simulink model "vehicleModel"  (R2022a)
settings: Solver=VariableStepAuto  StartTime=0  StopTime=20  FixedStep=0.01  RelTol=1e-3
InitFcn:
  | lat_sim_parameters
values from neighbouring files (symbols this model uses):
  A = zeros(6)    [find_path_coeffs.m]    (also in getLateralDynamics.m = [0 1 vx 0)
  B = [0; -b1; 0; -b2]    [getLateralDynamics.m]
  C = [1 0 d 0]    [lat_sim_parameters.m]
  Klat = place(A, B, poles)    [lat_sim_parameters.m]    (also in tuneLateralController.m)
  lr = 1.6    [acc_sim_parameters.m]    (also in lat_sim_parameters.m = 2; tuneLateralController.m = 2)
  m = 1575    [acc_sim_parameters.m]    (also in lat_sim_parameters.m = 2000; tuneLateralController.m = 2000)
undefined symbols (not defined in the file or in its folder): vxBar
libraries: autolibshared x1
settings Model: Creator=Fernando VM  LastModifiedBy=fvall
settings SolverCC: AlgebraicLoopSolver=TrustRegion
settings DataIOCC: ExternalInput=[dt, da, dd]  ReturnWorkspaceOutputs=off
settings DebuggingCC: UnconnectedInputMsg=warning  UnconnectedOutputMsg=warning  UnconnectedLineMsg=warning  SFMachineParentedDataDiag=warning  ArithmeticOperatorsInVariantConditions=warning
settings SFSimCC: CustomCodeUndefinedFunction=UseInterfaceOnly

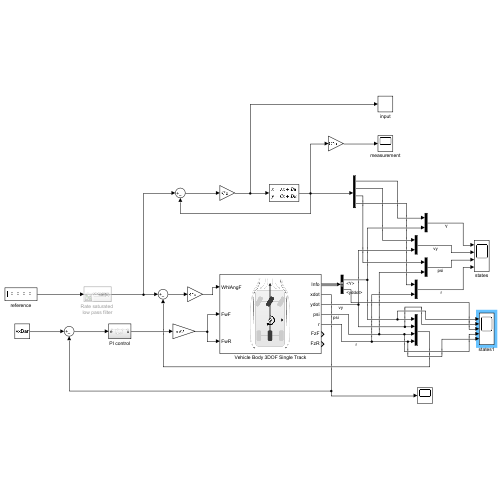
[thumbnail: Simulink's stored preview of the top-level diagram]
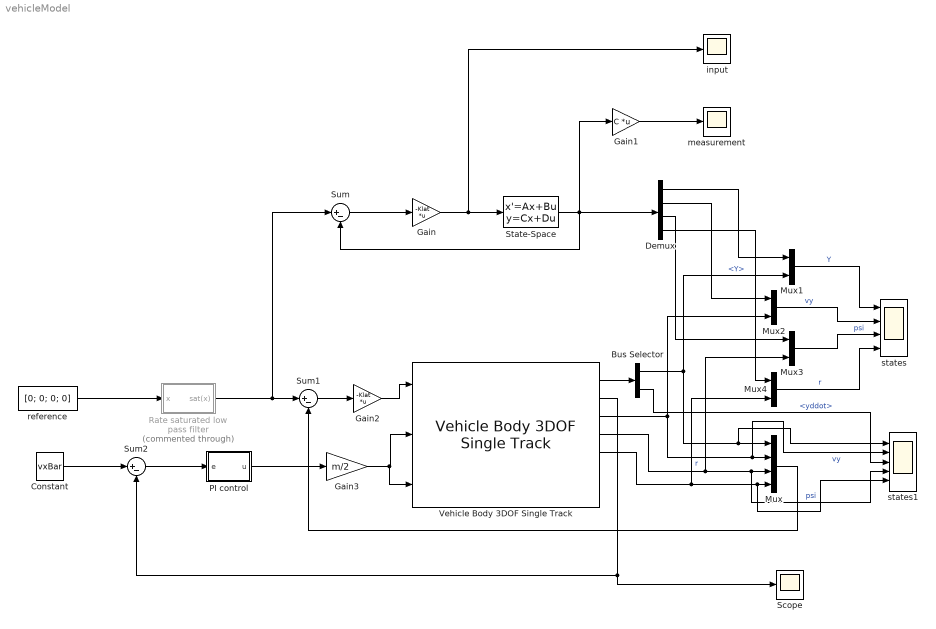
== system vehicleModel ==
  Bus Selector : BusSelector  OutputSignals=InertFrm.Cg.Disp.Y,BdyFrm.Cg.Acc.yddot
  Constant : Constant  Value=vxBar
  Demux : Demux
  Gain : Gain  Gain=-Klat  Multiplication=Matrix(K*u)
  Gain1 : Gain  Gain=C  Multiplication=Matrix(K*u)
  Gain2 : Gain  Gain=-Klat  Multiplication=Matrix(K*u)
  Gain3 : Gain  Gain=m/2
  Mux : Mux
  Mux{1..4} (4 alike) : Mux  Inputs=2
  PI control : Subsystem
  Rate saturated low pass filter : Subsystem  Commented=through
  Scope : Scope
  State-Space : StateSpace  A=A  B=B  C=eye(4)  D=zeros(4,1)  InitialCondition=[3.6; 0 ; 0; 0]
  Sum : Sum  Inputs=|+-
  Sum1 : Sum  Inputs=|+-
  Sum2 : Sum  Inputs=|+-
  Vehicle Body 3DOF Single Track : autolibshared/Vehicle Body 3DOF Single Track  trackMode=Single (bicycle)  inputMode=External longitudinal forces  frontSteerMode=on  rearSteerMode=off  windMode=off  muMode=off  extFMode=off  extMMode=off  htchFMode=off  htchMMode=off  extXo=off  extpsio=off  extxdoto=off  extro=off  extYo=off  extTamb=off  extydoto=off  aMode=2  NF=2  NR=2  m=m  a=lf  b=lr  h=0.35  dh=1  hh=0.2  X_o=0  xdot_o=vxBar  CalphaMode=off  sigmaMode=on  d=0  hl=0  w=[1.4,1.4]  Cy_f=CfReal  Cy_r=CrReal  sigma_f=.1  sigma_r=.1  alpha_f_brk=[-.1 .1]  Cy_f_data=[-9e3 9e3]  alpha_r_brk=[-.1 .1]  Cy_r_data=[-9e3 9e3]  Y_o=3.6  ydot_o=0  Izz=4000  psi_o=0  r_o=0  Af=2  Cd=.3  Cl=.1  Cpm=.1  beta_w=[0:0.01:0.3]  Cs=[0:0.03:0.9]  Cym=[0:0.01:0.3]  Pabs=101325  Tair=273  g=9.81  mu=1  xdot_tol=.01  Fznom=5000  Fxtire_sat=7e4  Fytire_sat=7e4  longOff=0  latOff=0  vertOff=0  wrapAng=off
      settings: SourceProductBaseCode=PW,DR,MT,VE
  input : Scope
  measurement : Scope
  reference : Constant  Value=[0; 0; 0; 0]
  states : Scope  NumInputPorts=4
  states1 : Scope  NumInputPorts=5
  wires:
  Gain1/1 -> measurement/1
  Gain/1 -> input/1, State-Space/1
  State-Space/1 -> Gain1/1, Sum/2, Demux/1
  Sum/1 -> Gain/1
  Demux/1 -> Mux1/1
  Sum1/1 -> Gain2/1
  Gain2/1 -> Vehicle Body 3DOF Single Track/1
  Vehicle Body 3DOF Single Track/1 -> Bus Selector/1
  Bus Selector/1 -> states1/1, Mux/1, Mux1/2  "<Y>"
  Vehicle Body 3DOF Single Track/3 -> Mux2/2, states1/2, Mux/2  "vy"
  Vehicle Body 3DOF Single Track/4 -> Mux3/2, states1/4, Mux/3  "psi"
  Vehicle Body 3DOF Single Track/5 -> Mux4/2, states1/5, Mux/4  "r"
  Mux/1 -> Sum1/2
  Mux1/1 -> states/1  "Y"
  Demux/2 -> Mux2/1
  Demux/3 -> Mux3/1
  Demux/4 -> Mux4/1
  Mux2/1 -> states/2  "vy"
  Mux3/1 -> states/3  "psi"
  Mux4/1 -> states/4  "r"
  Gain3/1 -> Vehicle Body 3DOF Single Track/3, Vehicle Body 3DOF Single Track/2
  Constant/1 -> Sum2/1
  Vehicle Body 3DOF Single Track/2 -> Scope/1, Sum2/2
  Bus Selector/2 -> states1/3  "<yddot>"
  Sum2/1 -> PI control/1(e)
  PI control/1(u) -> Gain3/1
  Rate saturated low pass filter/1(sat(x)) -> Sum/1, Sum1/1
  reference/1 -> Rate saturated low pass filter/1(x)

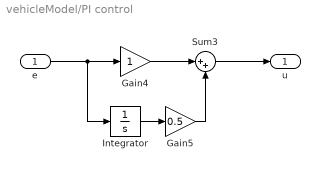
== system vehicleModel/PI control ==
  e : Inport
  Gain4 : Gain
  Gain5 : Gain  Gain=0.5
  Integrator : Integrator
  Sum3 : Sum  Inputs=|++
  u : Outport  VectorParamsAs1DForOutWhenUnconnected=off
  wires:
  e/1 -> Gain4/1, Integrator/1
  Sum3/1 -> u/1
  Gain4/1 -> Sum3/1
  Integrator/1 -> Gain5/1
  Gain5/1 -> Sum3/2

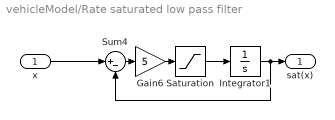
== system vehicleModel/Rate saturated low pass filter ==
  x : Inport
  Gain6 : Gain  Gain=5
  Integrator1 : Integrator  InitialCondition=[3.6 0 0 0]
  Saturation : Saturate  UpperLimit=2  LowerLimit=-2
  Sum4 : Sum  Inputs=|+-
  sat(x) : Outport  VectorParamsAs1DForOutWhenUnconnected=off
  wires:
  Sum4/1 -> Gain6/1
  Gain6/1 -> Saturation/1
  Saturation/1 -> Integrator1/1
  x/1 -> Sum4/1
  Integrator1/1 -> Sum4/2, sat(x)/1
